simulink model "pendulo_resorte_"  (R2025a)
settings: Solver=FixedStepAuto  StartTime=0.0  StopTime=10.0  FixedStep=4e-3  RelTol=1e-3
settings Model: Creator=Control Room  LastModifiedBy=Control Room

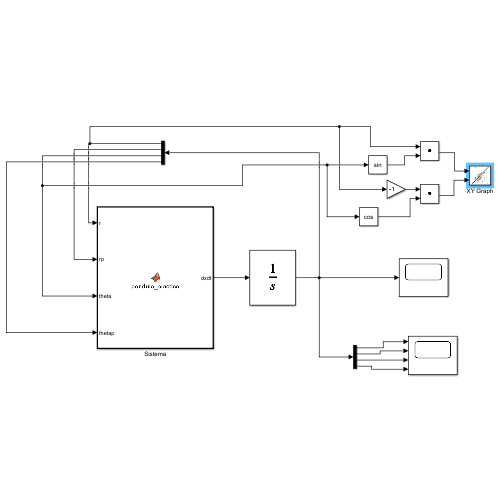
[thumbnail: Simulink's stored preview of the top-level diagram]
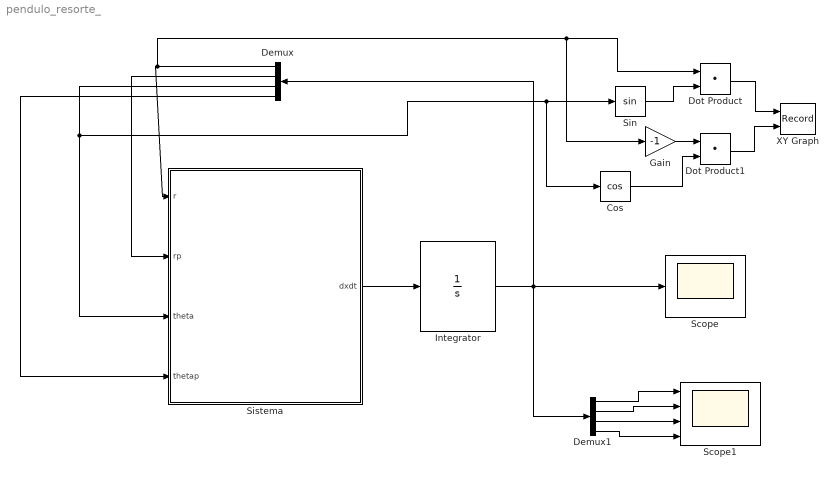
== system pendulo_resorte_ ==
  Cos : Trigonometry  Operator=cos
  Demux : Demux
  Demux1 : Demux
  Dot Product : DotProduct  OutDataTypeStr=Inherit: Inherit via internal rule
  Dot Product1 : DotProduct  OutDataTypeStr=Inherit: Inherit via internal rule
  Gain : Gain  Gain=-1
  Integrator : Integrator  InitialCondition=[0.7; 0; pi/6; 0];
  Scope : Scope
      settings: ActiveDisplayYMinimum=-3.559385761724688  ActiveDisplayYMaximum=3.5762041126406987
  Scope1 : Scope  NumInputPorts=4
      settings: ActiveDisplayYMinimum=0.40089788094381607  ActiveDisplayYMaximum=0.79829790979256454
  Sin : Trigonometry
  Sistema : MATLAB Function  TreatAsAtomicUnit=on
  XY Graph : Record  NumPorts=2.0  FileSettingsInternal="{\"entries\":[{\"content\":{\"excelSettings\":{\"content\":{},\"type\":\"Streamout.ExcelSettings\"},\"parquetSettings\":{\"content\":{},\"type\":\"Streamout.ParquetSettings\"}},\"type\":\"Streamout.FileSettingStorage\",\"uuid\":\"\"}],\"packageUris\":[\"http:\\/\\/schema.mathworks.com\\/mf0\\/streamout_blocks\\/R2020a\"],\"version\":\"1.0\"}"  FrameSettings=[0, 0]  Layout=[1 1]  SignalsInternal="{\"entries\":[{\"content\":{\"signals\":[{\"content\":{\"blockPath\":[],\"dimensions\":[1],\"domain\":\"\",\"lineColor\":\"#a2142f\",\"plots\":[ 1 ],\"port\":1,\"sid\":[\"\"],\"signalID\":1,\"signalName\":\"Dot Product\"},\"type\":\"RecordBlkView.Signal\",\"uuid\":\"\"},{\"content\":{\"blockPath\":[],\"dimensions\":[1],\"domain\":\"\",\"lineColor\":\"#139fff\",\"plots\":[ 1 ],\"port\":2,\"sid\":[\"\"],\"signalID\":2,\"signalName\":\"Dot Product1\"},\"type\":\"RecordBlkView.Signal\",\"uuid\":\"\"}]},\"type\":\"RecordBlkView.InputSignals\",\"uuid\":\"\"}],\"packageUris\":[\"http:\\/\\/schema.mathworks.com\\/mf0\\/streamout_blocks\\/R2020a\"],\"version\":\"1.0\"}"  VisualizationBindings="{\"xyplotplugin\":{\"info\":[{\"series\":[{\"bindingParametersList\":[{\"parameter\":\"X-Axis\",\"signalID\":1,\"signalName\":\"Dot Product\"},{\"parameter\":\"Y-Axis\",\"signalID\":2,\"signalName\":\"Dot Product1\"}],\"seriesID\":0}],\"subplotID\":1}]}}"  CompatibilityTag=XY
  wires:
  Sistema/1(dxdt) -> Integrator/1
  Integrator/1 -> Demux1/1, Scope/1, Demux/1
  Demux/1 -> Gain/1, Dot Product/1, Sistema/1(r)
  Demux/2 -> Sistema/2(rp)
  Demux/3 -> Sistema/3(theta), Cos/1, Sin/1
  Demux/4 -> Sistema/4(thetap)
  Demux1/1 -> Scope1/1
  Demux1/2 -> Scope1/2
  Demux1/3 -> Scope1/3
  Demux1/4 -> Scope1/4
  Sin/1 -> Dot Product/2
  Dot Product/1 -> XY Graph/1
  Gain/1 -> Dot Product1/1
  Cos/1 -> Dot Product1/2
  Dot Product1/1 -> XY Graph/2

== matlab function pendulo_resorte_/Sistema ==
  data: r input; dxdt output; rp input; theta input; thetap input
function dxdt = pendulo_elastico(r,rp,theta,thetap)
    m=10;
    l=0.5;
    k=1000;
    g=9.8;
    %X(1)=r X(2)=rp X(3)=theta X(4)=thetap
    X = [r rp theta thetap];
    x1p=X(2);
    x3p=X(4);
    x2p=g*cos(X(3))-(k/m)*(X(1)-l)+ X(1)*X(4)^2;
    x4p=-(2*X(2)*X(4)+g*sin(X(3)))/X(1);
    dxdt=[x1p; x2p; x3p; x4p;];
